simulink model "sim_nonlinear_pend"  (R2024a)
settings: Solver=ode4  StartTime=0.0  StopTime=SIMULATION_TIME  FixedStep=STEP_SIZE  RelTol=1e-3
values from neighbouring files (symbols this model uses):
  a1 = identified_para.a1    [dd_sim_linearSys_oneshot.m]    (also in dd_sim_nonlinearSys.m; dd_simulation.m; dd_simulation_itr.m; sim_linearSys_itr.m)
  a2 = identified_para.a2    [dd_sim_linearSys_oneshot.m]    (also in dd_sim_nonlinearSys.m; dd_simulation.m; dd_simulation_itr.m; sim_linearSys_itr.m)
  b1 = identified_para.b1    [dd_sim_linearSys_oneshot.m]    (also in dd_sim_nonlinearSys.m; dd_simulation.m; dd_simulation_itr.m; sim_linearSys_itr.m)
  b2 = identified_para.b2    [dd_sim_linearSys_oneshot.m]    (also in dd_sim_nonlinearSys.m; dd_simulation.m; dd_simulation_itr.m; sim_linearSys_itr.m)
  g = 9.81    [dd_sim_linearSys_oneshot.m]    (also in dd_sim_nonlinearSys.m; dd_simulation.m; dd_simulation_itr.m; sim_linearSys_itr.m)
  K = Kip1    [dd_initialization.m]    (also in dd_main.m = [10 1 1 -0.1]; dd_sim_linearSys_oneshot.m = [10 1 10 1]; dd_sim_nonlinearSys.m = [10 1 10 1]; exp_Conclusion.m = R \ B' * P0)
  L1 = 9.20e-02    (= 0.092)    [dd_sim_linearSys_oneshot.m]    (also in dd_sim_nonlinearSys.m; dd_simulation.m; dd_simulation_itr.m; sim_linearSys_itr.m)
  x0 = [0.920542212035 -4.28141076583 -0.0163775001355 -1.46742275595]    [K0_2407081823.mat]    (also in dd_main.m = dd_x(:,1); dd_main_solution.m = zeros(size(A,1),1); dd_sim_linearSys_oneshot.m = [-2 0 0 0]'; dd_sim_nonlinearSys.m = [2 0 1 0]')
settings Model: Creator=Huan  LastModifiedBy=Huan

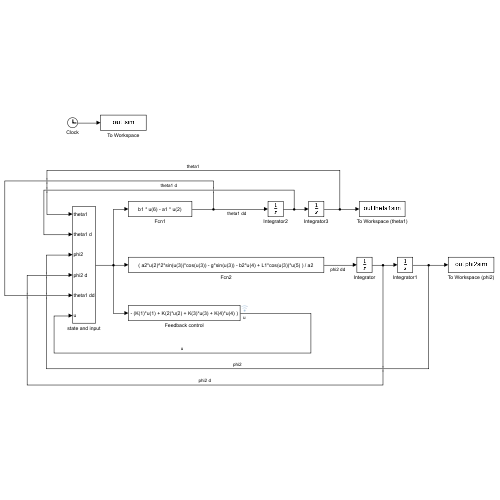
[thumbnail: Simulink's stored preview of the top-level diagram]
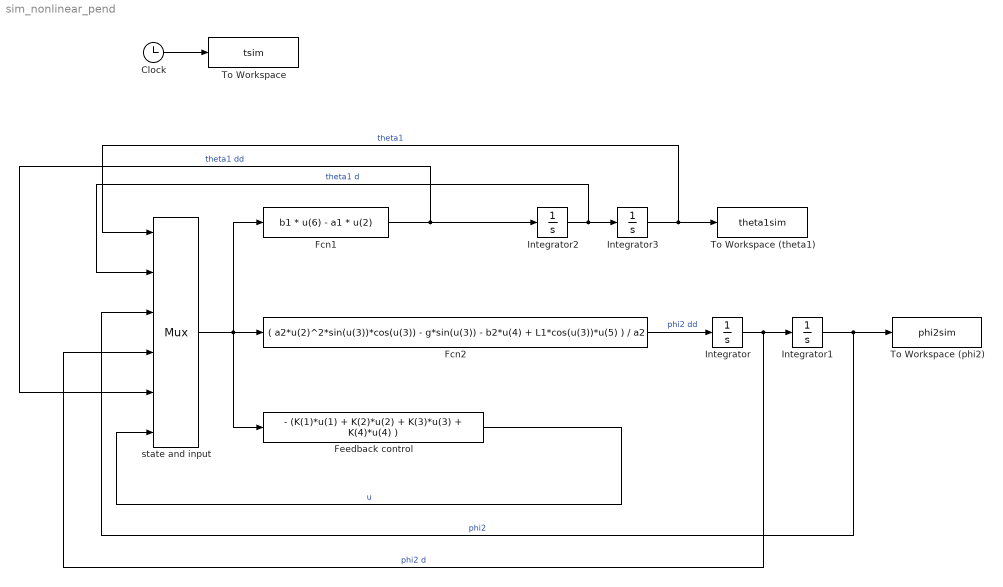
== system sim_nonlinear_pend ==
  Clock : Clock
  Fcn1 : Fcn  Expr=b1 * u(6) - a1 * u(2)
  Fcn2 : Fcn  Expr=( a2*u(2)^2*sin(u(3))*cos(u(3)) - g*sin(u(3)) - b2*u(4) + L1*cos(u(3))*u(5) ) / a2
  Feedback control : Fcn  Expr=- (K(1)*u(1) + K(2)*u(2) + K(3)*u(3) + K(4)*u(4) )
  Integrator : Integrator  InitialCondition=x0(4)
  Integrator1 : Integrator  InitialCondition=x0(3)
  Integrator2 : Integrator  InitialCondition=x0(2)
  Integrator3 : Integrator  InitialCondition=x0(1)
  To Workspace : ToWorkspace  VariableName=tsim  SampleTime=-1
  To Workspace (phi2) : ToWorkspace  VariableName=phi2sim  SampleTime=-1
  To Workspace (theta1) : ToWorkspace  VariableName=theta1sim  SampleTime=-1
  state and input : Mux  Inputs=6
      settings: DisplayOption=signals
  wires:
  Integrator1/1 -> To Workspace (phi2)/1, state and input/3  "phi2"
  Fcn2/1 -> Integrator/1  "phi2 dd"
  Integrator/1 -> Integrator1/1, state and input/4  "phi2 d"
  Clock/1 -> To Workspace/1
  Integrator2/1 -> Integrator3/1, state and input/2  "theta1 d"
  Fcn1/1 -> state and input/5, Integrator2/1  "theta1 dd"
  Integrator3/1 -> state and input/1, To Workspace (theta1)/1  "theta1"
  state and input/1 -> Fcn1/1, Fcn2/1, Feedback control/1
  Feedback control/1 -> state and input/6  "u"
